simulink subsystem "Inverter"  (R2022b)
settings: Solver=VariableStepAuto  StartTime=0.0  StopTime=10.0  RelTol=1e-3
values from neighbouring files (symbols this model uses):
  eps_i = motor.noload_current*1e-3    [BLDCmotor.m]
  Vs = motor.Vs    [BLDCmotor.m]    (also in geraModeloHover.m = 36)
settings Model: Creator=hemil  LastModifiedBy=hemil
settings OptimizationCC: ReuseModelBlockBuffer=on

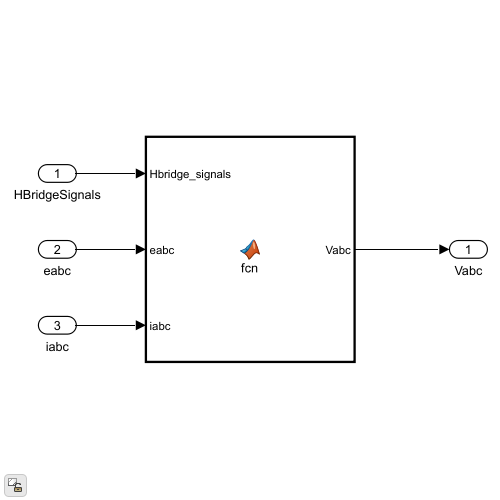
[thumbnail: Simulink's stored preview of the top-level diagram]
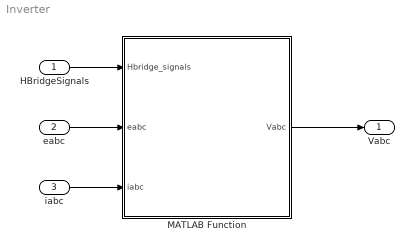
== system Inverter ==
  HBridgeSignals : Inport
  eabc : Inport  Port=2
  iabc : Inport  Port=3
  MATLAB Function : MATLAB Function  TreatAsAtomicUnit=on
  Vabc : Outport
  wires:
  HBridgeSignals/1 -> MATLAB Function/1(Hbridge_signals)
  MATLAB Function/1(Vabc) -> Vabc/1
  eabc/1 -> MATLAB Function/2(eabc)
  iabc/1 -> MATLAB Function/3(iabc)

== matlab function Inverter/MATLAB Function ==
  data: Hbridge_signals input; eabc input; iabc input; Vs parameter; Vabc output; eps_i parameter
function Vabc  = fcn(Hbridge_signals, eabc, iabc, Vs, eps_i)    
    % Compute phase voltages based on H-bridge signals
    Va = voltCalc(Hbridge_signals(1), eabc(1), iabc(1), Vs, eps_i); % Va calculation
    Vb = voltCalc(Hbridge_signals(2), eabc(2), iabc(2), Vs, eps_i); % Vb calculation
    Vc = voltCalc(Hbridge_signals(3), eabc(3), iabc(3), Vs, eps_i); % Vc calculation

    Vabc = [Va Vb Vc]';
end

function V = voltCalc(H, e, i, Vs, eps_i)
    if H == 1
        V = Vs;
    elseif H == -1
        V = 0;
    else
        if i > eps_i
            V = 0;  % Current is flowing to the motor, so clamped to 0V
        elseif i < -eps_i
            V = Vs; % Current is flowing back to the inverter, so clamped to Vs
        else % abs(i) < esp_i
            V = e; % If the current is very small, assume the voltage holds steady
        end
    end
end
